simulink model "BLDCSym"  (R2022b)
settings: Solver=FixedStepAuto  StartTime=0.0  StopTime=Tend  RelTol=1e-3
values from neighbouring files (symbols this model uses):
  J_m = J_w    (= 0.00701)    [BLDCmotor.m]
  Kf = motor.Kf    [BLDCmotor.m]    (also in geraModeloHover.m = 0.0150833220093)
settings Model: Creator=hemil  LastModifiedBy=hemil
settings OptimizationCC: ReuseModelBlockBuffer=on
settings RTWCC: GenerateReport=on  LaunchReport=on

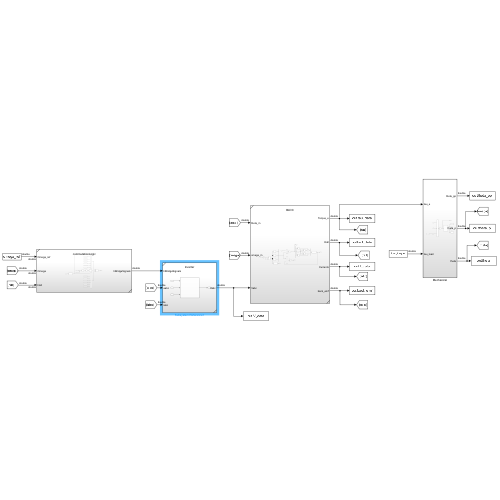
[thumbnail: Simulink's stored preview of the top-level diagram]
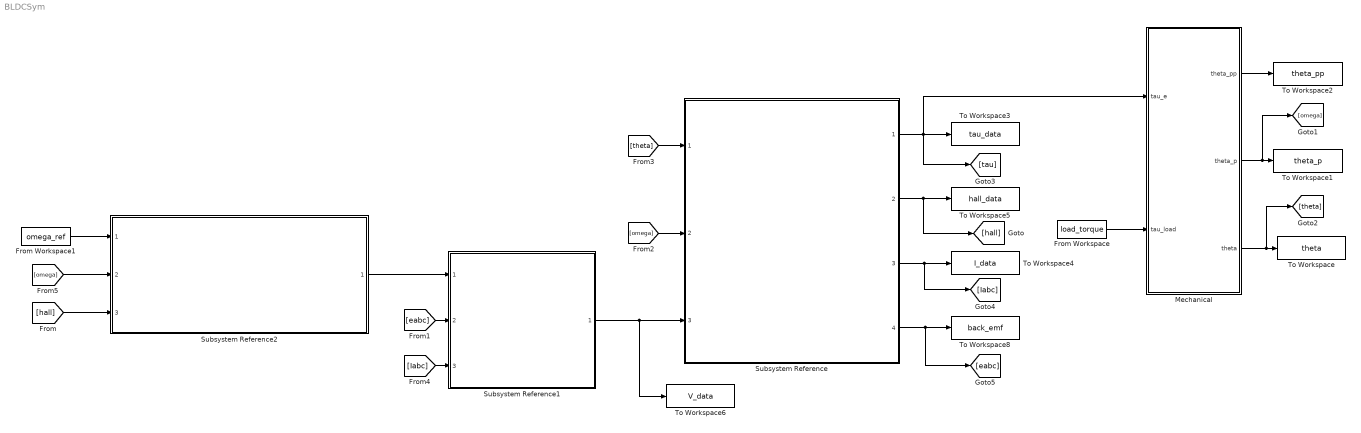
== system BLDCSym ==
  From Workspace : FromWorkspace  VariableName=load_torque
  From Workspace1 : FromWorkspace  VariableName=omega_ref
  Mechanical : Subsystem
  Subsystem Reference : Subsystem  ReferencedSubsystem=BLDC
  Subsystem Reference1 : Subsystem  ReferencedSubsystem=Inverter
  Subsystem Reference2 : Subsystem  ReferencedSubsystem=commutationLogic
  To Workspace : ToWorkspace  VariableName=theta  SampleTime=-1
      settings: Save2DSignal=2-D array (concatenate along first dimension)
  To Workspace1 : ToWorkspace  VariableName=theta_p  SampleTime=-1
      settings: Save2DSignal=2-D array (concatenate along first dimension)
  To Workspace2 : ToWorkspace  VariableName=theta_pp  SampleTime=-1
      settings: Save2DSignal=2-D array (concatenate along first dimension)
  To Workspace3 : ToWorkspace  VariableName=tau_data  SampleTime=-1
      settings: Save2DSignal=2-D array (concatenate along first dimension)
  To Workspace4 : ToWorkspace  VariableName=I_data  SampleTime=-1
  To Workspace5 : ToWorkspace  VariableName=hall_data  SampleTime=-1
  To Workspace6 : ToWorkspace  VariableName=V_data  SampleTime=-1
  To Workspace8 : ToWorkspace  VariableName=back_emf  SampleTime=-1
  wires:
  Subsystem Reference/2 -> [hall], To Workspace5/1
  Subsystem Reference/1 -> Mechanical/1(tau_e), [tau], To Workspace3/1
  Mechanical/2(theta_p) -> [omega], To Workspace1/1
  [omega] -> Subsystem Reference/2
  Mechanical/3(theta) -> [theta], To Workspace/1
  [theta] -> Subsystem Reference/1
  Mechanical/1(theta_pp) -> To Workspace2/1
  Subsystem Reference/3 -> [Iabc], To Workspace4/1
  From Workspace/1 -> Mechanical/2(tau_load)
  Subsystem Reference/4 -> [eabc], To Workspace8/1
  Subsystem Reference1/1 -> To Workspace6/1, Subsystem Reference/3
  [eabc] -> Subsystem Reference1/2
  [Iabc] -> Subsystem Reference1/3
  Subsystem Reference2/1 -> Subsystem Reference1/1
  [hall] -> Subsystem Reference2/3
  [omega] -> Subsystem Reference2/2
  From Workspace1/1 -> Subsystem Reference2/1

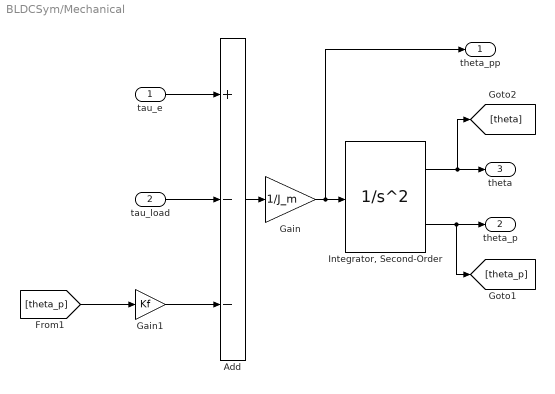
== system BLDCSym/Mechanical ==
  tau_e : Inport
  tau_load : Inport  Port=2
  Add : Sum  Inputs=+--
  Gain : Gain  Gain=1/J_m
  Gain1 : Gain  Gain=Kf
  "Integrator, Second-Order" : SecondOrderIntegrator  ICDXDT=0
  theta_pp : Outport
  theta_p : Outport  Port=2
  theta : Outport  Port=3
  wires:
  [theta_p] -> Gain1/1
  Add/1 -> Gain/1
  Gain/1 -> "Integrator, Second-Order"/1, theta_pp/1
  tau_e/1 -> Add/1
  "Integrator, Second-Order"/1 -> [theta], theta/1
  "Integrator, Second-Order"/2 -> [theta_p], theta_p/1
  Gain1/1 -> Add/3
  tau_load/1 -> Add/2
